simulink model "sistema"  (R2023b)
settings: Solver=VariableStepAuto  StartTime=0.0  StopTime=10.0  RelTol=1e-3
settings Model: Creator=marco  LastModifiedBy=marco
settings DataIOCC: SaveOutput=off  SignalLogging=off  DSMLogging=off  ReturnWorkspaceOutputs=off  TimeSaveName=t
settings DebuggingCC: AlgebraicLoopMsg=none  ArtificialAlgebraicLoopMsg=none  MaxConsecutiveZCsMsg=none

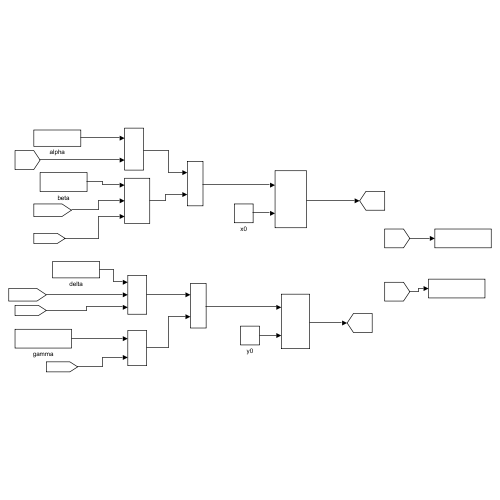
[thumbnail: Simulink's stored preview of the top-level diagram]
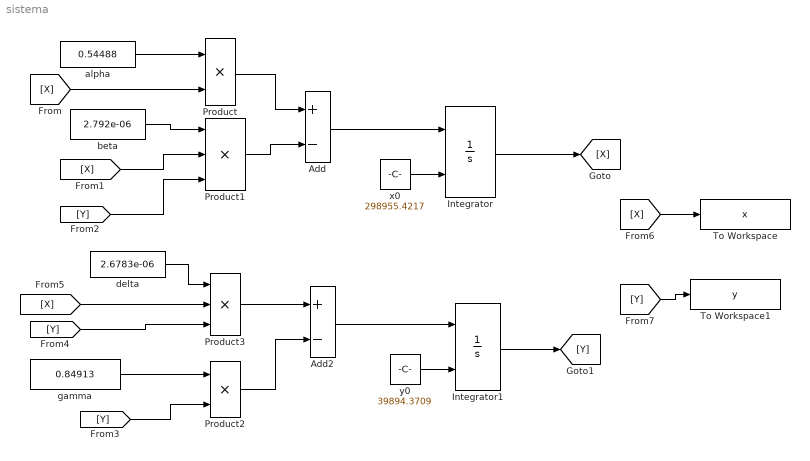
== system sistema ==
  Add : Sum  Inputs=+-
  Add2 : Sum  Inputs=+-
  Integrator : Integrator  InitialConditionSource=external
  Integrator1 : Integrator  InitialConditionSource=external
  Product : Product
  Product1 : Product  Inputs=3
  Product2 : Product
  Product3 : Product  Inputs=3
  To Workspace : ToWorkspace  VariableName=x  SampleTime=-1
  To Workspace1 : ToWorkspace  VariableName=y  SampleTime=-1
  alpha : Constant  Value=0.54488
  beta : Constant  Value=2.792e-06
  delta : Constant  Value=2.6783e-06
  gamma : Constant  Value=0.84913
  x0 : Constant  Value=298955.4217
  y0 : Constant  Value=39894.3709
  wires:
  x0/1 -> Integrator/2
  y0/1 -> Integrator1/2
  Add/1 -> Integrator/1
  Product1/1 -> Add/2
  Product/1 -> Add/1
  Add2/1 -> Integrator1/1
  Product3/1 -> Add2/1
  Product2/1 -> Add2/2
  gamma/1 -> Product2/1
  delta/1 -> Product3/1
  beta/1 -> Product1/1
  alpha/1 -> Product/1
  [X] -> Product/2
  Integrator/1 -> [X]
  [X] -> Product1/2
  Integrator1/1 -> [Y]
  [Y] -> Product1/3
  [Y] -> Product2/2
  [Y] -> Product3/3
  [X] -> Product3/2
  [X] -> To Workspace/1
  [Y] -> To Workspace1/1
